simulink model "ex1_HW4_Boeru"  (R2017b)
settings: Solver=FixedStepAuto  StartTime=0.0  StopTime=0.0006  FixedStep=0.0000002  RelTol=1e-3
settings Model: Creator=Iva  LastModifiedBy=Briana

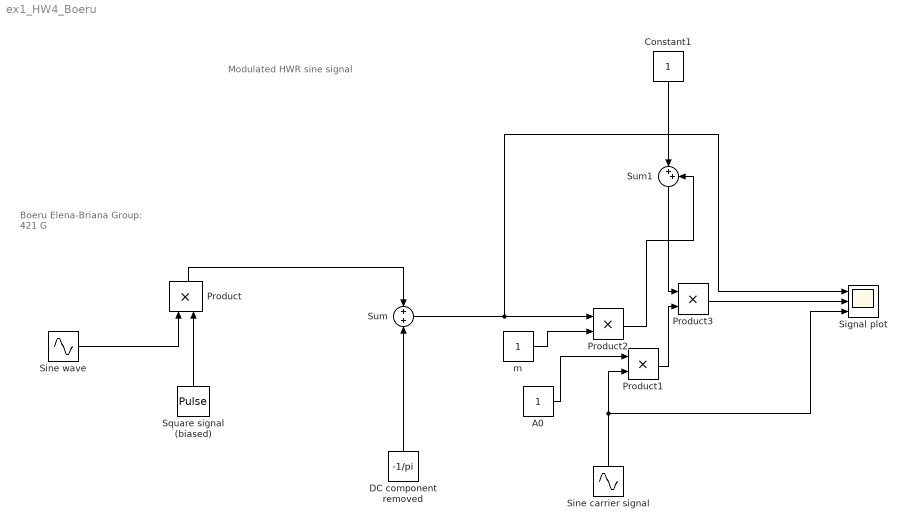
== system ex1_HW4_Boeru ==
  note: Boeru Elena-Briana
      | Group: 421 G
  note: Modulated HWR sine signal
  " DC component removed" : Constant  Value=-1/pi
  "A0 " : Constant
  Constant1 : Constant
  Product{,1..3} (4 alike) : Product
  Signal plot : Scope  NumInputPorts=3
  "Sine carrier signal " : Sin  Frequency=2*pi*500000  SampleTime=0
  Sine wave : Sin  Frequency=2*pi*5000  SampleTime=0
  "Square signal (biased) " : DiscretePulseGenerator  PulseType=Time based  Period=0.0002  PulseWidth=50
  Sum : Sum  Inputs=2
  Sum1 : Sum  Inputs=|++
  m : Constant
  wires:
  Sine wave/1 -> Product/1
  " DC component removed"/1 -> Sum/2
  Product/1 -> Sum/1
  Sum/1 -> Product2/1, Signal plot/1
  m/1 -> Product2/2
  Product2/1 -> Sum1/2
  Constant1/1 -> Sum1/1
  Sum1/1 -> Product3/1
  Product1/1 -> Product3/2
  "A0 "/1 -> Product1/1
  "Sine carrier signal "/1 -> Signal plot/3, Product1/2
  "Square signal (biased) "/1 -> Product/2
  Product3/1 -> Signal plot/2
